simulink model "Tetraedro_model_sem_sim_com_FK"  (R2013a)
settings: Solver=ode4  StartTime=0.0  StopTime=1000  FixedStep=.05  MaxStep=0.05  RelTol=1e-3
libraries: aerolibutil x3, vrlib x2, aerolibtransform2 x1, instrumentlib x1
settings Model: Creator=Daniel  LastModifiedBy=Administrator

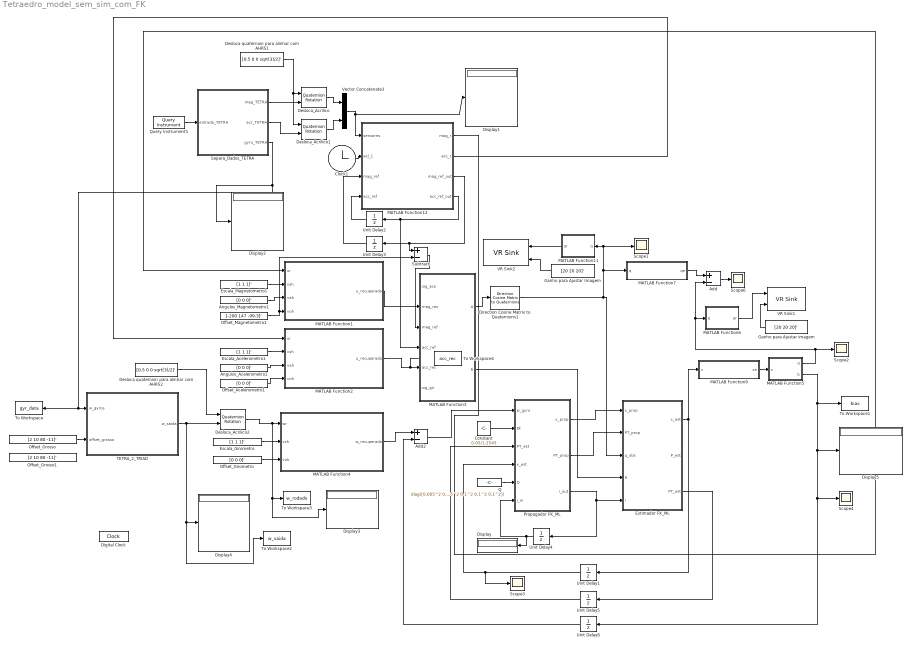
== system Tetraedro_model_sem_sim_com_FK ==
  Add : Sum  Inputs=+-
  Add2 : Sum  Inputs=+-
  Angulos_Acelerometro1 : Constant  Value=[0 0 0]'
  Angulos_Magnetometro1 : Constant  Value=[0 0 0]'
  Clock1 : Clock
  Constant : Constant  Value=0.05/1.2545
  Desloca quaternion para alinhar com AHRS1 : Constant  Value=[0.5 0 0 sqrt(3)/2]'
  Desloca quaternion para alinhar com AHRS2 : Constant  Value=[0.5 0 0 sqrt(3)/2]'
  Desloca_Acrilico : aerolibutil/Quaternion Rotation
  Desloca_Acrilico1 : aerolibutil/Quaternion Rotation
  Desloca_Acrilico2 : aerolibutil/Quaternion Rotation
  Digital Clock : DigitalClock
  Direction Cosine Matrix to Quaternions1 : aerolibtransform2/Direction Cosine Matrix  to Quaternions
  Display{,1..5} (6 alike) : Display
      Display1 settings: Format=binary (Stored Integer)
      Display2 settings: Format=binary (Stored Integer)
      Display3 settings: Format=binary (Stored Integer)
      Display4 settings: Format=binary (Stored Integer)
      Display5 settings: Format=binary (Stored Integer)
  Escala_Acelerometro1 : Constant  Value=[1 1 1]'
  Escala_Girometro : Constant  Value=[1 1 1]'
  Escala_Magnetometro1 : Constant  Value=[1 1 1]'
  Estimador FK_ML : MATLAB Function  TreatAsAtomicUnit=on
  Ganho para Ajustar Imagem : Constant  Value=[20 20 20]'
  Ganho para Ajustar imagem : Constant  Value=[20 20 20]'
  MATLAB Function1 : MATLAB Function  TreatAsAtomicUnit=on
  MATLAB Function11 : MATLAB Function  TreatAsAtomicUnit=on
  MATLAB Function12 : MATLAB Function  TreatAsAtomicUnit=on
  MATLAB Function2 : MATLAB Function  TreatAsAtomicUnit=on
  MATLAB Function3 : MATLAB Function  TreatAsAtomicUnit=on
  MATLAB Function4 : MATLAB Function  TreatAsAtomicUnit=on
  MATLAB Function5 : MATLAB Function  TreatAsAtomicUnit=on
  MATLAB Function6 : MATLAB Function  TreatAsAtomicUnit=on
  MATLAB Function7 : MATLAB Function  TreatAsAtomicUnit=on
  MATLAB Function9 : MATLAB Function  TreatAsAtomicUnit=on
  Offset_Acelerometro1 : Constant  Value=[0 0 0]'
  Offset_Girometro : Constant  Value=[0 0 0]'
  Offset_Grosso : Constant  Value=[2 10 80 -11]'
  Offset_Grosso1 : Constant  Value=[2 10 80 -11]'
  Offset_Magnetometro1 : Constant  Value=[-200 147 -99.3]'
  Propagador FK_ML : MATLAB Function  TreatAsAtomicUnit=on
  Q : Constant  Value=diag([0.005^2 0.005^2 0.005^2 0.1^2 0.1^2 0.1^2])
  Query Instrument1 : instrumentlib/Query Instrument  sampleTime=.05  isWorkspaceObject=off  timeout=5  inputBufferSize=200  protocol=Serial  serialPort=COM3  baudRate=115200  gpibVendor=Advantech  boardIndex=0  primaryAddress=1  secondaryAddress=0  visaVendor=Agilent  visaSerialPort=0  chassisIndex=0  logicalAddress=0  tcpRemoteHost='127.0.0.1'  tcpRemotePort=4500  udpRemoteHost='127.0.0.1'  udpRemotePort=9090  visaTCPBoardIndex=0  visaTCPRemoteHost='127.0.0.1'  usbBoardIndex=0  usbManufID=0  usbModelCode=0  usbSerialNumber=0  initAction=None  initCommand='DATA:SOURCE CH1'  initFunction=get  queryCommand='#'  responseFormat=ASCII  asciiFormatting='%d %d %d %d %d %d %d %f %d %f %d %f %d %f'  precision=16-bit integer  byteOrder=Little endian  valuesToRead=18  removeBytes=on  afterOutputAction=Repeat query for new data  enableFrames=on  frameSize=14
  Scope{1..4,6} (5 alike) : Scope
      Scope1 settings: TimeRange=1000  YMin=-0.008  YMax=0.013  SaveName=ScopeData2  MaxDataPoints=50000
      Scope2 settings: TimeRange=1000  YMin=-0.008  YMax=0.013  SaveName=ScopeData3  MaxDataPoints=50000
      Scope3 settings: YMin=-1  YMax=1  MaxDataPoints=60000
      Scope4 settings: TimeRange=1000  YMin=-0.008  YMax=0.013  SaveName=ScopeData4  MaxDataPoints=50000
      Scope6 settings: TimeRange=1000  YMin=-0.0125  YMax=0.015  MaxDataPoints=50000
  Separa_Dados_TETRA : MATLAB Function  TreatAsAtomicUnit=on
  Subtract : Sum  Inputs=+-
  TETRA_2_TRIAD : MATLAB Function  TreatAsAtomicUnit=on
  To Workspace : ToWorkspace  VariableName=gyr_data  SampleTime=-1
  To Workspace1 : ToWorkspace  VariableName=bias  SampleTime=-1
  To Workspace2 : ToWorkspace  VariableName=w_saida  SampleTime=-1
  To Workspace3 : ToWorkspace  VariableName=w_rodado  SampleTime=-1
  To Workspace4 : ToWorkspace  VariableName=acc_rec  SampleTime=-1
  Unit Delay1 : UnitDelay  InitialCondition=[0 0 0 1 0 0 0]'  SampleTime=-1
  Unit Delay2 : UnitDelay  InitialCondition=[0 0 0]'  SampleTime=-1
  Unit Delay3 : UnitDelay  InitialCondition=[0 0 0]'  SampleTime=-1
  Unit Delay4 : UnitDelay  SampleTime=-1
  Unit Delay5 : UnitDelay  InitialCondition=diag([1 1 1 1 1 1])*1E6  SampleTime=-1
  Unit Delay6 : UnitDelay  InitialCondition=[0 0 0]'  SampleTime=-1
  VR Sink1 : vrlib/VR Sink  InstantiateOnLoad=on  SampleTime=-1  ViewEnable=on  RemoteChange=off  RemoteView=off  FieldsWritten=H.rotation.4.1.1.double#H.scale.3.1.1.double  WorldFileName=C:\Users\Administrator\Desktop\Arquivos WRL\teste_combinado2.wrl  AutoView=off  VideoDimensions=[]  AllowVariableSize=off
  VR Sink2 : vrlib/VR Sink  InstantiateOnLoad=on  SampleTime=-1  ViewEnable=on  RemoteChange=off  RemoteView=off  FieldsWritten=H.rotation.4.1.1.double#H.scale.3.1.1.double  WorldFileName=C:\Users\Administrator\Desktop\TCC Daniel\Arquivos WRL\teste_combinado.wrl  AutoView=off  VideoDimensions=[]  AllowVariableSize=off
  Vector Concatenate3 : Concatenate
  wires:
  Escala_Acelerometro1/1 -> MATLAB Function2/2(vsh)
  Angulos_Acelerometro1/1 -> MATLAB Function2/3(vah)
  Offset_Acelerometro1/1 -> MATLAB Function2/4(voh)
  Escala_Magnetometro1/1 -> MATLAB Function1/2(vsh)
  Angulos_Magnetometro1/1 -> MATLAB Function1/3(vah)
  MATLAB Function2/1(u_recuperado) -> To Workspace4/1, MATLAB Function3/5(acc_rec)
  MATLAB Function1/1(u_recuperado) -> MATLAB Function3/2(mag_rec)
  MATLAB Function3/1(A) -> Direction Cosine Matrix to Quaternions1/1
  Unit Delay2/1 -> MATLAB Function12/4(acc_ref)
  Unit Delay3/1 -> MATLAB Function12/3(mag_ref)
  MATLAB Function12/3(mag_ref_out) -> Subtract/1, Unit Delay3/1
  MATLAB Function12/4(acc_ref_out) -> Unit Delay2/1, MATLAB Function3/4(acc_ref)
  Clock1/1 -> MATLAB Function12/2(sel_1)
  MATLAB Function12/1(mag_r) -> MATLAB Function1/1(ur)
  MATLAB Function12/2(acc_r) -> MATLAB Function2/1(ur)
  Separa_Dados_TETRA/1(mag_TETRA) -> Desloca_Acrilico/2
  Separa_Dados_TETRA/2(acc_TETRA) -> Desloca_Acrilico1/2
  Desloca quaternion para alinhar com AHRS1/1 -> Desloca_Acrilico1/1, Desloca_Acrilico/1
  Desloca_Acrilico/1 -> Vector Concatenate3/1
  Desloca_Acrilico1/1 -> Vector Concatenate3/2
  Vector Concatenate3/1 -> Display1/1, MATLAB Function12/1(sensores)
  Subtract/1 -> MATLAB Function3/3(mag_ref)
  MATLAB Function11/1(qr) -> VR Sink2/1
  Ganho para Ajustar Imagem/1 -> VR Sink2/2
  Offset_Magnetometro1/1 -> Subtract/2, MATLAB Function1/4(voh)
  Query Instrument1/1 -> Separa_Dados_TETRA/1(entrada_TETRA)
  Escala_Girometro/1 -> MATLAB Function4/2(vsh)
  Offset_Girometro/1 -> MATLAB Function4/3(voh)
  MATLAB Function4/1(w_recuperado) -> Add2/1
  MATLAB Function5/2(b) -> Scope4/1, Unit Delay6/1, Display5/1, To Workspace1/1
  Propagador FK_ML/1(x_prop) -> Estimador FK_ML/1(x_prop)
  Propagador FK_ML/3(i_out) -> Unit Delay4/1, Estimador FK_ML/5(i)
  Unit Delay4/1 -> Display/1, Propagador FK_ML/6(i_in)
  Q/1 -> Propagador FK_ML/5(Q)
  Constant/1 -> Propagador FK_ML/2(Dt)
  MATLAB Function3/2(R) -> Estimador FK_ML/4(R)
  Estimador FK_ML/3(PT_est) -> Unit Delay5/1
  Unit Delay1/1 -> Scope3/1, Propagador FK_ML/4(x_est)
  Unit Delay5/1 -> Propagador FK_ML/3(PT_est)
  Propagador FK_ML/2(PT_prop) -> Estimador FK_ML/2(PT_prop)
  Estimador FK_ML/1(x_est) -> Unit Delay1/1, MATLAB Function9/1(x)
  Direction Cosine Matrix to Quaternions1/1 -> MATLAB Function11/1(q), Scope1/1, MATLAB Function7/1(q), Estimador FK_ML/3(q_obs)
  Add2/1 -> Propagador FK_ML/1(w_gyro)
  MATLAB Function9/1(xe) -> MATLAB Function5/1(x)
  MATLAB Function5/1(q) -> Scope2/1, Add/2, MATLAB Function6/1(q)
  Add/1 -> Scope6/1
  MATLAB Function7/1(qe) -> Add/1
  Ganho para Ajustar imagem/1 -> VR Sink1/2
  MATLAB Function6/1(qr) -> VR Sink1/1
  TETRA_2_TRIAD/1(w_saida) -> To Workspace2/1, Display4/1, Desloca_Acrilico2/2
  Separa_Dados_TETRA/3(gyro_TETRA) -> TETRA_2_TRIAD/1(w_gyros), To Workspace/1, Display2/1
  Offset_Grosso/1 -> TETRA_2_TRIAD/2(offset_grosso)
  Unit Delay6/1 -> Add2/2
  Desloca_Acrilico2/1 -> To Workspace3/1, Display3/1, MATLAB Function4/1(wr)
  Desloca quaternion para alinhar com AHRS2/1 -> Desloca_Acrilico2/1

== matlab function Tetraedro_model_sem_sim_com_FK/MATLAB Function1 ==
  data: ur input; u_recuperado output; vsh input; vah input; voh input
function u_recuperado = inv_triad_model(ur,vsh,vah,voh)
%#eml

rho = vah(1);
phi = vah(2);
lambda = vah(3);

T_inv = [1 0 0; -tan(rho) 1/cos(rho) 0;...
    tan(rho)*tan(lambda)-tan(phi) -tan(lambda)/cos(rho) 1/(cos(lambda)*cos(phi))];
S_inv = inv(diag(vsh));

u_recuperado = T_inv*S_inv*(ur - voh);

== matlab function Tetraedro_model_sem_sim_com_FK/TETRA_2_TRIAD ==
  data: w_gyros input; w_saida output; offset_grosso input
function w_saida  = Tetra_2_TRIAD(w_gyros, offset_grosso)
%#codegen

s_12 = w_gyros(4) - offset_grosso(4);
s_23 = w_gyros(3) - offset_grosso(3);
s_31 = w_gyros(2) - offset_grosso(2);
s_456 = w_gyros(1) - offset_grosso(1);

s_12 = s_12*0.2439*pi/180;
s_23 = s_23*0.2439*pi/180;
s_31 = s_31*0.2439*pi/180;
s_456 = s_456*0.2439*pi/180;

S = [s_12; s_23; s_31; s_456];

H = [0 2*sqrt(2)/3 1/3; -sqrt(6)/3 -sqrt(2)/3 1/3; ...
    sqrt(6)/3 -sqrt(2)/3 1/3; 0 0 -1];

w_saida = inv(H'*H)*H'*S;

== matlab function Tetraedro_model_sem_sim_com_FK/MATLAB Function11 ==
  data: q input; qr output
function qr = ajusta_q(q)
%#eml

q = q/(norm(q));
v = [q(2) q(3) q(4)] / norm([q(2) q(3) q(4)]);
ang = acos(q(1))*2;

qr = [v ang];

== matlab function Tetraedro_model_sem_sim_com_FK/MATLAB Function12 ==
  data: sensores input; sel_1 input; mag_r output; acc_r output; mag_ref input; acc_ref input; mag_ref_out output; acc_ref_out output
function [mag_r, acc_r, mag_ref_out, acc_ref_out] = fcn(sensores, sel_1, mag_ref, acc_ref)
%#codegen

mag_ref_out = zeros(3,1);
acc_ref_out = zeros(3,1);

mag_x = sensores(1);
mag_y = sensores(2);
mag_z = sensores(3);

acc_x = sensores(4);
acc_y = sensores(5);
acc_z = sensores(6);

mag_ref_out = mag_ref;
acc_ref_out = acc_ref;

if sel_1 == 0
mag_ref_out = [mag_x mag_y mag_z]';
acc_ref_out = [acc_x acc_y acc_z]';
end

mag_r = [mag_x mag_y mag_z]';
acc_r = [acc_x acc_y acc_z]';

== matlab function Tetraedro_model_sem_sim_com_FK/MATLAB Function2 ==
  data: ur input; u_recuperado output; vsh input; vah input; voh input
function u_recuperado = inv_triad_model(ur,vsh,vah,voh)
%#eml

rho = vah(1);
phi = vah(2);
lambda = vah(3);

T_inv = [1 0 0; -tan(rho) 1/cos(rho) 0;...
    tan(rho)*tan(lambda)-tan(phi) -tan(lambda)/cos(rho) 1/(cos(lambda)*cos(phi))];
S_inv = inv(diag(vsh));

u_recuperado = T_inv*S_inv*(ur - voh);

== matlab function Tetraedro_model_sem_sim_com_FK/MATLAB Function3 ==
  data: sig_ace input; A output; mag_rec input; mag_ref input; acc_ref input; acc_rec input; sig_gir input; R output
function [A,R] = TRIAD(sig_ace,mag_rec,mag_ref,acc_ref,acc_rec,sig_gir)

% ========== Função de Determinação de Atitude ===========
% ========== Algoritmo TRIAD ===========
% Os parâmetros de Entrada são:
% V1 : vetor de referência V1
V1 = acc_ref;
% V2 : vetor de referência V2
V2 = mag_ref;
% W1 : vetor de observação W1
W1 = acc_rec;
% W2 : vetor de observação W2
W2 = mag_rec;
% SigTo1 : desvio padrão das observação do Acelerômetro
SigTot1 = sig_ace;
% SigTo2 : desvio padrão das observação do Magnetômetro
SigTot2 = sig_gir;

% ========================================================
% Os parâmetros de Retorno são:
% A : matriz de atitude
% P : Covariância da atitude
% ========================================================
% --- Obtendo a Tríade de Referência
r1 = V1/norm(V1);
r2 = cross(V1,V2); % função do produto vetorial
r2 = r2 / norm(r2);
r3 = cross(r1,r2);
% --- Montando a Matriz de Referência
Mref = [r1 r2 r3];

% --- Obtendo a tríade de observação
s1 = W1/norm(W1);
s2 = cross(W1,W2);
s2 = s2 / norm(s2);
s3 = cross(s1,s2);
% --- Montando a Matriz de Observação
Mobs = [s1 s2 s3];
% --- Atitude pelo TRIAD
A = Mobs * Mref';
%--------------------------------------------------------------------------
% Obtendo a covariância da atitude (P = P + AP AT)
R = SigTot1^2 * eye(3) + ...
    (1/norm(cross(W1,W2)))^2 * (SigTot1^2* (W1'*W2) * (W1*W2' + W2*W1')...
    + (SigTot2^2 - SigTot1^2)*W1*W1');

%--------------------------------------------------------------------------

== matlab function Tetraedro_model_sem_sim_com_FK/Separa_Dados_TETRA ==
  data: mag_TETRA output; entrada_TETRA input; acc_TETRA output; gyro_TETRA output
function [mag_TETRA, acc_TETRA, gyro_TETRA]  = separa_dados(entrada_TETRA)
%#codegen

mag_TETRA = zeros(3,1);
acc_TETRA = zeros(3,1);
gyro_TETRA = zeros(4,1);

mag_x = entrada_TETRA(1);
mag_y = entrada_TETRA(2);
mag_z = entrada_TETRA(3);

acc_x = entrada_TETRA(4);
acc_y = entrada_TETRA(5);
acc_z = entrada_TETRA(6);

gyro_placa_1 = entrada_TETRA(7);
gyro_placa_2 = entrada_TETRA(9);
gyro_placa_3 = entrada_TETRA(11);
gyro_placa_4 = entrada_TETRA(13);

mag_TETRA = [mag_x mag_y mag_z]';
acc_TETRA = [acc_x acc_y acc_z]';
gyro_TETRA = [gyro_placa_1 gyro_placa_2 gyro_placa_3 gyro_placa_4]';

== matlab function Tetraedro_model_sem_sim_com_FK/MATLAB Function7 ==
  data: q input; qe output
function qe = tira_redundancia(q)
qe = zeros(4,1);
%#eml

 if q(1)<0.0
     qe = -q;
 else
    qe = q;
 end

== matlab function Tetraedro_model_sem_sim_com_FK/MATLAB Function4 ==
  data: wr input; w_recuperado output; vsh input; voh input
function w_recuperado = inv_gyro_model(wr,vsh,voh)
%#eml

S_inv = inv(diag(vsh));

w_recuperado = S_inv*(wr - voh);

== matlab function Tetraedro_model_sem_sim_com_FK/MATLAB Function9 ==
  data: x input; xe output
function xe = tira_redundancia(x)
xe = zeros(7,1);
 if (x(4)<0.0)
     xe(1:4,1) = -x(1:4,1);
     xe(5:7,1) = x(5:7,1);
 else
    xe = x;
 end

== matlab function Tetraedro_model_sem_sim_com_FK/MATLAB Function5 ==
  data: x input; q output; b output
function [q,b] = separa(x)
q = [x(4,1); x(1:3,1)];
b = x(5:7,1);
end

== matlab function Tetraedro_model_sem_sim_com_FK/MATLAB Function6 ==
  data: q input; qr output
function qr = ajusta_q(q)
%#eml

q = q/(norm(q));
v = [q(2) q(3) q(4)] / norm([q(2) q(3) q(4)]);
ang = acos(q(1))*2;

qr = [v ang];

== matlab function Tetraedro_model_sem_sim_com_FK/Propagador FK_ML ==
  data: w_gyro input; x_prop output; Dt input; PT_est input; x_est input; Q input; PT_prop output; i_in input; i_out output
function [x_prop, PT_prop, i_out] = propagador_FK(w_gyro, Dt, PT_est, x_est, Q, i_in)
%#codegen

i_out = i_in + 1;

% ================== Propagação ==================
% ------ Propagação do Estado
% São medidos os Girômetros e sua saída subtraida
% do bias é integrada no período de propagação

q_est = x_est(1:4,1);
b_est = x_est(5:7,1);


% Matriz de atualização do quaternion
Th = w_gyro * Dt;

Omega4 = [ 0     Th(3) -Th(2)  Th(1);
	  -Th(3)  0     Th(1)  Th(2); 
      Th(2) -Th(1)  0     Th(3);
     -Th(1) -Th(2) -Th(3)  0   ];

M = eye(4) * cos(norm(Th)/2) + Omega4 * sin(norm(Th)/2) / norm(Th);
q_prop = M * q_est; 

b_prop = b_est;

x_prop = [q_prop ; b_prop];

% Matriz Constante // A ser executado fora dessa função
GT = [ -1/2*eye(3) zeros(3,3); zeros(3,3) eye(3)];
QT = GT * Q * GT';

% ---------------------

Omega3_prop = [ 0     q_prop(3) -q_prop(2);
	  -q_prop(3)  0     q_prop(1); 
      q_prop(2) -q_prop(1)  0   ];

A_prop = (q_prop(4)^2 - norm(q_prop(1:3,1))^2)*eye(3) + 2*q_prop(1:3,1)*q_prop(1:3,1)' ... 
      + 2*q_prop(4)*Omega3_prop;
  
Omega3_est = [ 0     q_est(3) -q_est(2);
	  -q_est(3)  0     q_est(1); 
      q_est(2) -q_est(1)  0   ];  
  
A_est = (q_est(4)^2 - norm(q_est(1:3,1))^2)*eye(3) + 2*q_est(1:3,1)*q_est(1:3,1)' ... 
      + 2*q_est(4)*Omega3_est;
  
% ------ Propagação da Matriz de Covariância
L = A_prop * A_est';
KK = -1/2 * (L + eye(3)) * Dt/2;  % Integral Trapézio
PhiT = [L KK; zeros(3,3) eye(3)];
SiG = (PhiT * QT * PhiT' + QT) * Dt/2; % Integral Trapézio
PT_prop = PhiT * PT_est * PhiT' + SiG;

== matlab function Tetraedro_model_sem_sim_com_FK/Estimador FK_ML ==
  data: x_prop input size=7; x_est output size=7; PT_prop input size=[6,6]; q_obs input; R input; P_est output; PT_est output size=[6,6]; i input
function [x_est, P_est, PT_est] = Estimador_FK(x_prop, PT_prop, q_obs, R, i)

q = q_obs;
q_obs = [q(2); q(3); q(4); q(1)];

% ---- Separando as compoentes do estado
q_prop = x_prop(1:4,1);
b_prop = x_prop(5:7,1);


% ---- Montando a matriz E (Ksi)
E = [ q_prop(4) -q_prop(3)  q_prop(2);
      q_prop(3)  q_prop(4) -q_prop(1);
     -q_prop(2)  q_prop(1)  q_prop(4);
     -q_prop(1) -q_prop(2) -q_prop(3)];

% ---- Montando a matriz S
S  = [E zeros(4,3); zeros(3,3) eye(3)];

if (mod(i,50) ~= 0)    
    x_est = x_prop;
    PT_est = PT_prop;
    P_est   = S * PT_est * S';
else
    
% ---- Montando a matriz H e HT.
H  = [eye(4) zeros(4,3)];
HT = [E zeros(4,3)];

% ---- Separando covariancias dos estados
Ptt_prop = PT_prop(1:3,1:3);
Pbt_prop = PT_prop(4:6,1:3);

% ---- Cálculo do novo ganho (reduzido)
KT       = [Ptt_prop; Pbt_prop] * inv(Ptt_prop + R) * E';
% KT       = [Ptt_prop; Pbt_prop] * E' * inv(E*(Ptt_prop + P_Tri)*E');

    
% ---- Atualização da covariância reduzida
PT_est  = PT_prop - KT * HT * PT_prop; 

% ---- Cálculo da covariância estendida
P_est   = S * PT_est * S' ;

% ---- Cálculo do ganho estendido 
K        = S * KT;

% ---- Atualização do estado
if(dot(q_prop,q_obs) > 0)
    q_obs = q_obs;
else
    q_obs = -q_obs;
end

x_est   = x_prop + K * (q_obs - q_prop);

% ---- renormalização do quaternion
n = norm(x_est(1:4));           % norma do quatérnio
x_est(1:4,1) = x_est(1:4,1) / n; % renormalização do quaternion

end
